simulink model "qnorm_test1"  (Simulink 7.0)
settings: Solver=FixedStepDiscrete  StartTime=0.0  StopTime=stop_time  FixedStep=1.0  RelTol=1e-3
Description:
  | Timing Test: Quaternion Normalization, method 1
  | 
  | Copyright (c) 2001-2009, Jay A. St. Pierre.  All rights reserved.
settings Model: Creator=stpierre  LastModifiedBy=stpierre  ExtModeTrigMode=oneshot  ExtModeArmWhenConnect=off  ExtModeAutoUpdateStatusClock=off
settings DataIOCC: MaxDataPoints=1  SaveOutput=off  SaveTime=off
settings OptimizationCC: BlockReduction=off  BooleanDataType=off
settings DebuggingCC: SaveWithParameterizedLinksMsg=none  SignalResolutionControl=TryResolveAllWithWarning  SolverPrmCheckMsg=none  MultiTaskDSMMsg=warning  MultiTaskCondExecSysMsg=none  StrictBusMsg=None
settings HardwareCC: TargetUnknown=on
settings RTWCC: IncludeERTFirstTime=on

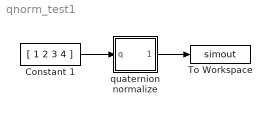
== system qnorm_test1 ==
  Constant 1 : Constant  Value=[ 1 2 3 4 ]
  To Workspace : ToWorkspace  VariableName=simout  SampleTime=-1  SaveFormat=Array
      settings: MaxDataPoints=1
  quaternion normalize : Subsystem
  wires:
  Constant 1/1 -> quaternion normalize/1(q)
  quaternion normalize/1(qnorm) -> To Workspace/1

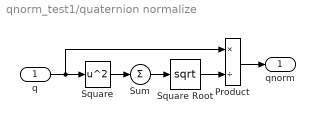
== system qnorm_test1/quaternion normalize ==
  q : Inport  PortDimensions=4
  Product : Product  Inputs=*/  SaturateOnIntegerOverflow=on  RndMeth=Zero  InputSameDT=on
  Square : Math  Operator=square  SaturateOnIntegerOverflow=on
  Square Root : Math  Operator=sqrt  SaturateOnIntegerOverflow=on
  Sum : Sum  Inputs=1  SaturateOnIntegerOverflow=on  InputSameDT=on
  qnorm : Outport  InitialOutput=0
  wires:
  Sum/1 -> Square Root/1
  Square/1 -> Sum/1
  q/1 -> Square/1, Product/1
  Square Root/1 -> Product/2
  Product/1 -> qnorm/1
